simulink library "ATM"  (R2016b)
settings: Solver=VariableStepAuto  StartTime=0.0  StopTime=10.0  RelTol=1e-3
libraries: aerolibatmos2 x1
settings Model: Creator=Andrew  LastModifiedBy=Andrew

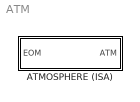
== system ATM ==
  ATMOSPHERE (ISA) : Subsystem

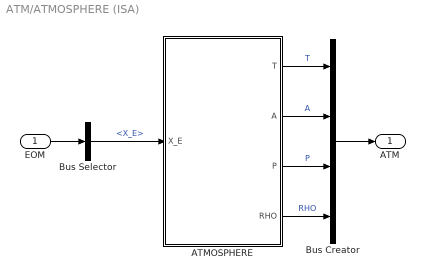
== system ATM/ATMOSPHERE (ISA) ==
  EOM : Inport
  ATMOSPHERE : Subsystem
  Bus Creator : BusCreator  Inputs=4
  Bus Selector : BusSelector  OutputSignals=X_E
  ATM : Outport
  wires:
  Bus Creator/1 -> ATM/1
  ATMOSPHERE/2(A) -> Bus Creator/2  "A"
  ATMOSPHERE/3(P) -> Bus Creator/3  "P"
  ATMOSPHERE/4(RHO) -> Bus Creator/4  "RHO"
  ATMOSPHERE/1(T) -> Bus Creator/1  "T"
  Bus Selector/1 -> ATMOSPHERE/1(X_E)  "<X_E>"
  EOM/1 -> Bus Selector/1

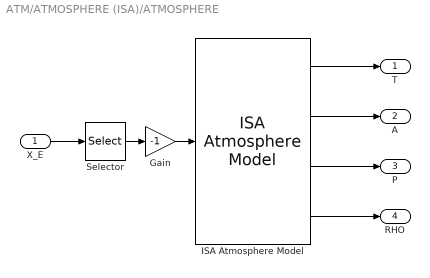
== system ATM/ATMOSPHERE (ISA)/ATMOSPHERE ==
  X_E : Inport
  Gain : Gain  Gain=-1
  ISA Atmosphere Model : aerolibatmos2/ISA Atmosphere Model  custom=on  g=9.80665  gamma=1.4  R=287.0531  L=0.0065  h_trop=11000  h_strat=20000  rho0=1.225  P0=101325  T0=288.15  h0=0
  Selector : Selector  InputPortWidth=3  IndexOptions=Index vector (dialog)  Indices=[3]  OutputSizes=1
  T : Outport
  A : Outport  Port=2
  P : Outport  Port=3
  RHO : Outport  Port=4
  wires:
  ISA Atmosphere Model/3 -> P/1
  ISA Atmosphere Model/1 -> T/1
  ISA Atmosphere Model/4 -> RHO/1
  ISA Atmosphere Model/2 -> A/1
  X_E/1 -> Selector/1
  Selector/1 -> Gain/1
  Gain/1 -> ISA Atmosphere Model/1
